simulink model "Model2"  (R2024b)
settings: Solver=ode4  StartTime=0.0  StopTime=100  FixedStep=0.01  RelTol=1e-3
values from neighbouring files (symbols this model uses):
  ARM_P_PID = [10 0 20]*0.1    [Single_ARM_Monte.m]    (also in main_starter.m)
  ARM_T_PID = [100 0 0]    [Single_ARM_Monte.m]    (also in main_starter.m)
  ARM_V_PID = [10 0 5]*0.1    [Single_ARM_Monte.m]    (also in main_starter.m)
  D_Joint0_angle0 = 45    [Single_ARM_Monte.m]    (also in main_starter.m)
  D_Joint0_angle1 = 0    [Single_ARM_Monte.m]    (also in main_starter.m)
  D_Joint0_angle2 = 0    [Single_ARM_Monte.m]    (also in main_starter.m)
  D_Joint0_rate0 = 0    [Single_ARM_Monte.m]    (also in main_starter.m)
  D_Joint0_rate1 = 0    [Single_ARM_Monte.m]    (also in main_starter.m)
  D_Joint0_rate2 = 0    [Single_ARM_Monte.m]    (also in main_starter.m)
  Joint_Motor_Mass = 23    [Single_ARM_Monte.m]    (also in main_starter.m)
  L_Joint0_angle0 = 45    [Single_ARM_Monte.m]    (also in main_starter.m)
  L_Joint0_angle1 = 0    [Single_ARM_Monte.m]    (also in main_starter.m)
  L_Joint0_angle2 = 0    [Single_ARM_Monte.m]    (also in main_starter.m)
  L_Joint0_rate0 = 0    [Single_ARM_Monte.m]    (also in main_starter.m)
  L_Joint0_rate1 = 0    [Single_ARM_Monte.m]    (also in main_starter.m)
  L_Joint0_rate2 = 0    [Single_ARM_Monte.m]    (also in main_starter.m)
  L_Joint_Offset = [ ... (first row only)    [Single_ARM_Monte.m]    (also in main_starter.m)
  Link1_Mass = 11    [Single_ARM_Monte.m]    (also in main_starter.m)
  Link2_Mass = 15.6    [Single_ARM_Monte.m]    (also in main_starter.m)
  Link3_Mass = 11    [Single_ARM_Monte.m]    (also in main_starter.m)
  Motor_transfer_Den = [1 100]    [Single_ARM_Monte.m]    (also in main_starter.m)
  Motor_transfer_Num = [100]    [Single_ARM_Monte.m]    (also in main_starter.m)
  PID_dt = 0.01    [Single_ARM_Monte.m]    (also in main_starter.m)
  R_Joint0_angle0 = 45    [Single_ARM_Monte.m]    (also in main_starter.m)
  R_Joint0_angle1 = 0    [Single_ARM_Monte.m]    (also in main_starter.m)
  R_Joint0_angle2 = 0    [Single_ARM_Monte.m]    (also in main_starter.m)
  R_Joint0_rate0 = 0    [Single_ARM_Monte.m]    (also in main_starter.m)
  R_Joint0_rate1 = 0    [Single_ARM_Monte.m]    (also in main_starter.m)
  R_Joint0_rate2 = 0    [Single_ARM_Monte.m]    (also in main_starter.m)
  RW_Att_D = 0.5    [Single_ARM_Monte.m]    (also in main_starter.m)
  RW_Att_I = 0.2    [Single_ARM_Monte.m]    (also in main_starter.m)
  RW_Att_P = 0.1    [Single_ARM_Monte.m]    (also in main_starter.m)
  RW_Mass = 100    [Single_ARM_Monte.m]    (also in main_starter.m)
  S_Body_Mass = 5    [Single_ARM_Monte.m]    (also in main_starter.m)
  S_init_pos = [0 0 0]'    [Single_ARM_Monte.m]    (also in main_starter.m)
  S_init_vel = [0 0 0]'    [Single_ARM_Monte.m]    (also in main_starter.m)
  T_Body_Mass = 4    [Single_ARM_Monte.m]    (also in main_starter.m)
  T_init_pos = [T_init_pos_list(i,1) T_init_pos_list(i,2) 0]'    [Single_ARM_Monte.m]    (also in main_starter.m = [1 0 0]')
  T_init_vel = [0 0 0]'    [Single_ARM_Monte.m]    (also in main_starter.m)
  Torq_mea_transfer_Den = [1 5]    [Single_ARM_Monte.m]    (also in main_starter.m)
  Torq_mea_transfer_Num = [5]    [Single_ARM_Monte.m]    (also in main_starter.m)
  U_Joint0_angle0 = 45    [Single_ARM_Monte.m]    (also in main_starter.m)
  U_Joint0_angle1 = 0    [Single_ARM_Monte.m]    (also in main_starter.m)
  U_Joint0_angle2 = 0    [Single_ARM_Monte.m]    (also in main_starter.m)
  U_Joint0_rate0 = 0    [Single_ARM_Monte.m]    (also in main_starter.m)
  U_Joint0_rate1 = 0    [Single_ARM_Monte.m]    (also in main_starter.m)
  U_Joint0_rate2 = 0    [Single_ARM_Monte.m]    (also in main_starter.m)
undefined symbols (not defined in the file or in its folder): X, Y, Z
libraries: nesl_utility x315, sm_lib x282, simulink_extras x46, sharedtransform x25, aerolibutil x4, simulink x2, matrix_library x2, dspmtrx3 x1
(part 11 of 12)

== matlab function Model2/Single(Right)_ARM_Simplify/touch ==
  settings: updateMethod=DISCRETE
  data: touch_start input; R_jtc input; R_Jd input; Rv_cmd input; speed_drop_flg output; touch_flg output; q_touch_flg output; speed_drop_vec output
function [speed_drop_flg, touch_flg, q_touch_flg, speed_drop_vec] = detectTouch3(touch_start, R_jtc, R_Jd, Rv_cmd)

    % --- 파라미터 설정 ---

    speed_err_thresh      = 1e-2;
    current_min_thresh    = 0.2e-3;
    current_max_thresh    = 2.5e-1;

    % --- 출력 초기화 ---
    speed_drop_flg  = 0;
    touch_flg       = 0;
    q_touch_flg     = 0;
    speed_drop_vec  = zeros(3,1);  % double 타입 고정

    % --- 전류 추출 ---
    R_qt0 = R_jtc(1);
    R_qt1 = R_jtc(2);
    R_qt2 = R_jtc(3);

    q0_touch_flg = 0;
    q1_touch_flg = 0;
    q2_touch_flg = 0;

    % --- 속도 차이 계산 ---
    raw_vec = abs(Rv_cmd - R_Jd) > speed_err_thresh;
    speed_drop_vec = double(raw_vec);  % 형 변환

    if any(raw_vec)
        speed_drop_flg = 1;
    end

    if touch_start == 1
        if abs(R_qt0) >= current_min_thresh && abs(R_qt0) < current_max_thresh
            q0_touch_flg = 1;
        end
        if abs(R_qt1) >= current_min_thresh && abs(R_qt1) < current_max_thresh
            q1_touch_flg = 1;
        end
        if abs(R_qt2) >= current_min_thresh && abs(R_qt2) < current_max_thresh
            q2_touch_flg = 1;
        end

        if q0_touch_flg || q1_touch_flg || q2_touch_flg
           touch_flg = 1;
        end

        % if  q_touch_flg
        %     touch_flg = 1;
        % end
    end
end

== matlab function Model2/Single(Right)_ARM_Simplify/MATLAB Function16 ==
  settings: updateMethod=DISCRETE
  data: R_J input; R_J_Pos input; R_q input; elapsedTime input; Body_f1 input; Body_f2 input; Body_f3 input; Body_f4 input; Z output; control_mode output; Rv_cmd output; flag_empty_now output; touch_start output; overload_start output; EE_Jaco_start output; system_empty input; system_overload input; system_slip_ing input; system_slip_confirm input; Body_contact output
function [Z,control_mode,Rv_cmd,flag_empty_now,touch_start,overload_start,EE_Jaco_start,Body_contact]  = mlhdlc_fsm_mealy(R_J, R_J_Pos, R_q, elapsedTime, ...
    Body_f1, Body_f2, Body_f3, Body_f4,system_empty,system_overload,system_slip_ing,system_slip_confirm) ...

% system_empty
% define states
S1 = 1; %% pre-grasping
S2 = 2; %% stay
S3 = 3; %% closing (grasping)
S4 = 4; %% regrasping_all
S5 = 5; %% grasp_complete


sub_overload = 11; %% regrasp_empty
sub_empty    = 22; %% regrasp_overload
sub_slip_ing = 33; %% regrasp_slip_ing
sub_slip_conf= 44; %% regrasp_slip_confirm



Rv_cmd = zeros(3,1);
control_mode = zeros(3,1);
flag_empty_now =0;
Z = zeros(1,1);

touch_start=0;
overload_start=0;
empty_start=0;
EE_Jaco_start=0;


% initial_R_condition = [-45 -5 -5];

persistent current_state
if isempty(current_state)
    current_state = 1;
end

persistent slip_latch
if isempty(slip_latch)
    slip_latch = 0;
end

persistent touch_start_flag
if isempty(touch_start_flag)
    touch_start_flag = 0;
end

persistent regrasp_substate
if isempty (regrasp_substate)
    regrasp_substate=0;
end

persistent grip_flg
if isempty(grip_flg)
    grip_flg = 0;
end

Body_contact = (Body_f1 && Body_f2 && Body_f3 && Body_f4) || ...
    (Body_f1 && Body_f3) || (Body_f2 && Body_f4);


%% FSM start

if current_state == S1

    % 
    R_condition_1 = (R_q(1) >= -45-2 && R_q(1) <= -45+2);
    R_condition_2 = (R_q(2) >= -5 && R_q(2) <= 5);
    R_condition_3 = (R_q(3) >= -5 && R_q(3) <= 5);

    R_condition = R_condition_1 && R_condition_2 && R_condition_3;

    condition = R_condition;
    % condition = 1;

    % Rv_cmd = [-45 0 0]'*pi/180;
    Rv_cmd = [-45 0 0]'*pi/180;
    control_mode = [3 3 3]';

    if (condition)
        if trackTime(elapsedTime, condition,1) >= 10
            current_state = 2;

            trackTime(elapsedTime, 0,1);
        end
    else
        current_state = 1;
    end

end

%%%%%%%%%%%%%%%%%%%%%%%%%%%%%%%%%%%%%%%%%%%%%%%%%%%%%%
%%%%%%%%%%%%%%%%%%%%%%%%%%%%%%%%%%%%%%%%%%%%%%%%%%%%%%

if current_state == S2


    if trackTime(elapsedTime, 1, 2) >= 10
        current_state = 3;
        trackTime(elapsedTime, 0, 2);
    else
        current_state = 2;
        Rv_cmd = [0 0 0]'*pi/180;
        control_mode = [2 2 2]';

    end
end

%%%%%%%%%%%%%%%%%%%%%%%%%%%%%%%%%%%%%%%%%%%%%%%%%%%%%%
%%%%%%%%%%%%%%%%%%%%%%%%%%%%%%%%%%%%%%%%%%%%%%%%%%%%%%

if current_state == S3 %% closing

    % Rv_cmd = [0.5 2 1.5]'*1*pi/180;

    Rv_cmd = [1 4 3]'*1*pi/180;
    control_mode = [2 2 2]';
    closing_duration = trackTime(elapsedTime,1,3);


    %%%%%%%%%%%%Predicate 활성화

    overload_start =1;
    empty_start =1;

    if closing_duration >= 5
        touch_start_flag = 1;
    end
    touch_start = touch_start_flag;

    %%%%%%%%%%%%Fail state

    if system_empty ==1 || system_overload==1 || system_slip_ing==1 || system_slip_confirm==1


        if system_empty == 1
            regrasp_substate = sub_empty;

        elseif system_overload == 1
            regrasp_substate = sub_overload;

        elseif system_slip_ing == 1
            regrasp_substate = sub_slip_ing;

        elseif system_slip_confirm == 1
            regrasp_substate = sub_slip_conf;

        end

        current_state = 4;

    end

    %%%%%%%%%%%%%%%%%%%%%%%

    if Body_contact == 1
        grasped_time = trackTime(elapsedTime, 1,4);

        if grasped_time>=1
            current_state = 2;
            trackTime(elapsedTime, 0,4);
        end
    else
        trackTime(elapsedTime, 0,4);
    end

else
    touch_start = 0;

end


%%%%%%%%%%%%%%%%%%%%%%%%%%%%%%%%%%%%%%%%%%%%%%%%%%%%%%
%%%%%%%%%%%%%%%%%%%%%%%%%%%%%%%%%%%%%%%%%%%%%%%%%%%%%%


if current_state == 4

    overload_start =1;
    empty_start =1;
    touch_start =1;
    EE_Jaco_start=1;

    if regrasp_substate == sub_empty

        Rv_cmd = [-1 -2 -1.5]'*pi/180;
        control_mode = [2 2 2]';

        R_condition_1 = (R_q(1) >= -28-2 && R_q(1) <= -28+2);
        R_condition_2 = (R_q(2) >= -2 && R_q(2) <= 2);
        R_condition_3 = (R_q(3) >= -2 && R_q(3) <= 2);

    
        if R_condition_1 && R_condition_2 && R_condition_3
            Rv_cmd = [0 0 0]'*pi/180;
            control_mode = [2 2 2]';
        end

    elseif regrasp_substate == sub_overload

        Rv_cmd = [-0.25 -1 -0.75]'*pi/180;
        control_mode = [2 2 2]';

    elseif regrasp_substate == sub_slip_ing

        Rv_cmd = [0.25 1 0.75]'*pi/180;
        control_mode = [2 2 2]';

        if system_slip_confirm == 1
            slip_latch = 1;  % 한 번이라도 잡히면 latch
        end

        if slip_latch == 1
            Rv_cmd = [-2 -4 -3]'*pi/180;
            control_mode = [2 2 2]';
            % slip_latch = 0;  
        end
        % 
        % elseif system_empty ==1
        %     regrasp_substate =sub_empty;
        % elseif system_overload ==1
        %     regrasp_substate = sub_overload;
        % end


    % elseif regrasp_substate == sub_slip_conf
    % 
    %     Rv_cmd = [-0.25 -1 -0.75]'*pi/180;
    %     control_mode = [2 2 2]';


    else
        Rv_cmd = [-3 -4 -3]';
        control_mode = [2 2 2]';
    end

    if Body_contact == 1
        grasped_time = trackTime(elapsedTime, 1,5);

        if grasped_time>=1
            current_state = 5;
            trackTime(elapsedTime, 0,5);
        end
    else
        trackTime(elapsedTime, 0,5);
    end

    % if some_recovery_condition
    %     current_state = S3;
    %     regrasp_substate = subS_none;
    % end

end


if current_state == 5

    overload_start =1;
  
    %
    % Rv_cmd = [2 4 5]'*pi/180;
    control_mode = [2 2 2]';
    EE = [R_J_Pos(1,4), R_J_Pos(2,4)]';
    EE_ = EE / norm(EE);

    Rv_cmd = [0 0 0]';
    

    if Body_contact == 1


        if grip_flg == 0
            grip_flg = 1;
            v_cmd = [-0.01; 0.0] .* EE_;
            R_Jacob = jacobian_3link(R_J);
            Rv_cmd = pinv(R_Jacob) * v_cmd;
        else
            Rv_cmd = [-2; -4; -3] * pi/180;
        end

        if (grip_flg == 1)
            v_cmd = [-0.01, 0.0]'.*EE_;
            R_Jacob = jacobian_3link(R_J);
            Rv_cmd = pinv(R_Jacob)*v_cmd;
        end

        % if system_overload == 1
        %     Rv_cmd = [-1; -2; -1];
        %     control_mode = [2 2 2]';
        %     return;
        % end

    end

   
end

  Z = current_state;

end


function J = jacobian_3link(theta)
% 링크 길이
L1 = 0.2;
L2 = 0.15;
L3 = 0.1;

t1 = theta(1);
t2 = theta(2);
t3 = theta(3);

t12 = t1 + t2;
t123 = t12 + t3;

% 자코비안 계산
J = zeros(2, 3);

J(1,1) = -L1*sin(t1) - L2*sin(t12) - L3*sin(t123);
J(1,2) =           - L2*sin(t12) - L3*sin(t123);
J(1,3) =                         - L3*sin(t123);

J(2,1) =  L1*cos(t1) + L2*cos(t12) + L3*cos(t123);
J(2,2) =             L2*cos(t12) + L3*cos(t123);
J(2,3) =                         L3*cos(t123);
end



function [temp] = trackTime(elapsedTime, timer_flg, id)
persistent isTiming startTime totalDuration
temp = 0;

if isempty(isTiming)
    isTiming = false(10,1);  % 최대 10개의 타이머 ID 지원
    startTime = zeros(10,1);
    totalDuration = zeros(10,1);
end


if timer_flg == 1 && ~isTiming(id)
    startTime(id) = elapsedTime;
    isTiming(id) = true;


elseif timer_flg == 1 && isTiming(id)
    currentDuration = elapsedTime - startTime(id);
    temp = currentDuration;


elseif timer_flg == 0 && isTiming(id)
    totalDuration(id) = elapsedTime - startTime(id);

    isTiming(id) = false;
    startTime(id) = 0;
    totalDuration(id) = 0;
end
end


%%%%%%%%%%%%%%

== matlab function Model2/Single_ARM/MATLAB Function5 ==
  data: v_sig input; v_out output; vd_out output; vd_sig input; t_mea input
function [v_out, vd_out] = limit_checker(v_sig,vd_sig,  t_mea)


if(abs(t_mea)>=0.5)
    vd_out = 0;
    v_out = 0;
else
    vd_out = vd_sig;
    v_out = v_sig;
end




end

== matlab function Model2/Single_ARM/MATLAB Function6 ==
  settings: updateMethod=DISCRETE
  data: cmd input; t_cmd output; cmd_d input; t_mea input; vd_mea input; v_mea input; p_mea input; mode input; tc_gain input; vc_gain input; pc_gain input; dt input
function t_cmd = motor_control(cmd,cmd_d, t_mea, vd_mea, v_mea, p_mea, mode, tc_gain, vc_gain, pc_gain, dt)

persistent I_save
persistent first_flg

if isempty(first_flg)
    I_save = 0;
    first_flg = 1;
end

if(mode == 1)%torque control
    % cmd : torque command [Nm]
    kp = tc_gain(1);
    ki = tc_gain(2);
    err = cmd - t_mea;
    t_cmd = kp*(cmd - t_mea) + ki*I_save;
    I_save = I_save + err*dt;

elseif(mode == 2) %velocity control
    % cmd : velocity command [rad/s]
    kp = vc_gain(1);
    % ki = vc_gain(2);
    kd = vc_gain(3);

    err = cmd - v_mea;
    errd = cmd_d - vd_mea;
    % t_cmd = (kp*err) + (kd*errd);
    t_cmd = (kp*err) + (kd*errd);
elseif(mode == 3) %position control : position command [rad]
    kp = pc_gain(1);
    % ki = pc_gain(2);
    kd = pc_gain(3);

    err = cmd - p_mea;
    errd = cmd_d - v_mea;
    t_cmd = (kp*err) + (kd*errd);
else%torque control
    t_cmd = 0;
end



end

== matlab function Model2/Single_ARM/MATLAB Function7 ==
  data: v_sig input; v_out output; vd_out output; vd_sig input; t_mea input
function [v_out, vd_out] = limit_checker(v_sig,vd_sig,  t_mea)


if(abs(t_mea)>=0.5)
    vd_out = 0;
    v_out = 0;
else
    vd_out = vd_sig;
    v_out = v_sig;
end




end

== matlab function Model2/Single(Right)_ARM_Simplify/slip_kinematics ==
  data: EE_vel_t output; EE_vel_J input; slip_kinematics output; EE_vel_J_pre input; EE_Jaco_start input
function [EE_vel_t,slip_kinematics]  = kinema_slip(EE_vel_J,EE_vel_J_pre,EE_Jaco_start)

    vel_min = -0.005;
    vel_max = 0.005;
    
    dvel_min = -0.005;
    dvel_max = 5e-03;
    
    dt= 3;
    
    dEE_vel = EE_vel_J_pre-EE_vel_J;
    EE_vel_t = dEE_vel/dt;
    
    if EE_Jaco_start==1 && all(EE_vel_J >= vel_min & EE_vel_J <= vel_max) && all(EE_vel_t<=dvel_max)
        slip_kinematics =1;
    else
        slip_kinematics=0;
    
    end

end

%%

== matlab function Model2/Single(Right)_ARM_Simplify/MATLAB Function1 ==
  data: u input; y output
function y = fcn(u)

y = u(:,3);

end

== matlab function Model2/Quad_ARM_Simplify/Mount_Frame_Based_Jacobian_Test/MATLAB Function4 ==
  data: u input; y output
function y = fcn(u)

y = u(:,4);

end

== matlab function Model2/Quad_ARM_Simplify/Mount_Frame_Based_Jacobian_Test/Right_ARM_Real_Simple_FK ==
  data: theta input; positions output; ee_pose output
function [positions, ee_pose] = fk_R_3link_simplify(theta)
    % theta: [theta1, theta2, theta3] (rad)
    % a1, a2, a3: 링크 길이
    % positions: [P0; P1; P2; P3] (각 조인트 위치)
    % ee_pose: [x, y, phi] (EE 위치 + 자세)
    % L0 = 0.04494;
    % L1 = 0.08979;
    % L2 = 0.1665;
    % L3a = 0.02945;
    % L3b = 0.1232;


    offset0 = -atan2(0.04494, 0.08979);
    offset1 = +atan2(0.04494, 0.08979);
    offset2 = -atan2(0.02945, 0.1232);
    offset = 1*[offset0,offset1,offset2]';

    theta = theta + offset;

    L = [sqrt(0.04494^2 + 0.08979^2);
           0.1665;
           sqrt(0.02945^2 + 0.1232^2)];

    theta1 = theta(1);
    theta2 = theta(2);
    theta3 = theta(3);

    % 누적 각도
    t1 = theta1;
    t2 = theta1 + theta2;
    t3 = t2 + theta3;

    % 각 조인트 위치 계산
    P0 = [0; 0];
    P1 = P0 + L(1) * [cos(t1); sin(t1)];
    P2 = P1 + L(2) * [cos(t2); sin(t2)];
    P3 = P2 + L(3) * [cos(t3); sin(t3)];

    % 자세
    phi = t3;

    % 출력
    positions = [P0, P1, P2, P3];  % 각 열이 각 위치
    ee_pose = [P3(1), P3(2)]'; % EE 위치 및 방향
end

== matlab function Model2/Quad_ARM_Simplify/Right_ARM_Real_FK ==
  data: theta input; positions output; ee_pose output
function [positions, ee_pose] = fk_R_3link_explicit(theta)
    L0 = 0.04494;
    L1 = 0.08979;
    L2 = 0.1665;
    L3a = 0.02945;
    L3b = 0.1232;

    t0 = theta(1);
    t1 = theta(2);
    t2 = theta(3);
    t01 = t0 + t1;
    t012 = t01 + t2;

    R = @(theta) [-cos(theta); -sin(theta)];

    P0 = [0; 0];
    P1 = P0 - L0 * R(t0 - pi/2);
    P2 = P1 - L1 * R(t0);
    P3 = P2 - L2 * R(t01);
    P4 = P3 - L3a * R(t012 - pi/2);
    ee_pose = P4 - L3b * R(t012);  % EE 위치
    positions = [P1,P2,P3,P4,ee_pose];
end

== matlab function Model2/Quad_ARM_Simplify/Right_ARM_Real_Simple_FK ==
  data: theta input; positions output; ee_pose output
function [positions, ee_pose] = fk_R_3link_simplify(theta)
    % theta: [theta1, theta2, theta3] (rad)
    % a1, a2, a3: 링크 길이
    % positions: [P0; P1; P2; P3] (각 조인트 위치)
    % ee_pose: [x, y, phi] (EE 위치 + 자세)
    % L0 = 0.04494;
    % L1 = 0.08979;
    % L2 = 0.1665;
    % L3a = 0.02945;
    % L3b = 0.1232;


    offset0 = -atan2(0.04494, 0.08979);
    offset1 = +atan2(0.04494, 0.08979);
    offset2 = -atan2(0.02945, 0.1232);
    offset = 1*[offset0,offset1,offset2]';

    theta = theta + offset;

    L = [sqrt(0.04494^2 + 0.08979^2);
           0.1665;
           sqrt(0.02945^2 + 0.1232^2)];

    theta1 = theta(1);
    theta2 = theta(2);
    theta3 = theta(3);

    % 누적 각도
    t1 = theta1;
    t2 = theta1 + theta2;
    t3 = t2 + theta3;

    % 각 조인트 위치 계산
    P0 = [0; 0];
    P1 = P0 + L(1) * [cos(t1); sin(t1)];
    P2 = P1 + L(2) * [cos(t2); sin(t2)];
    P3 = P2 + L(3) * [cos(t3); sin(t3)];

    % 자세
    phi = t3;

    % 출력
    positions = [P0, P1, P2, P3];  % 각 열이 각 위치
    ee_pose = [P3(1), P3(2)]'; % EE 위치 및 방향
end

== matlab function Model2/Quad_ARM_Simplify/MATLAB Function4 ==
  data: u input; y output
function y = fcn(u)

y = u(:,4);

end

== matlab function Model2/Quad_ARM_Simplify/Mount_Frame_Based_Jacobian_Test/Right_ARM_Jacobian ==
  data: theta input; J output
function J = jacobian_fk_R_3link_explicit(theta)
    % 링크 길이
    L0 = 0.04494;
    L1 = 0.08979;
    L2 = 0.1665;
    L3a = 0.02945;
    L3b = 0.1232;

    % 조인트 각도
    t0 = theta(1);
    t1 = theta(2);
    t2 = theta(3);

    t01 = t0 + t1;
    t012 = t01 + t2;

    % 편미분 벡터 함수 dR = d/dθ of R(θ)
    dR = @(theta) [sin(theta); -cos(theta)];

    % ∂x/∂theta1
    J1 = ...
        L0 * dR(t0 - pi/2) + ...
        L1 * dR(t0) + ...
        L2 * dR(t01) + ...
        L3a * dR(t012 - pi/2) + ...
        L3b * dR(t012);

    % ∂x/∂theta2
    J2 = ...
        L2 * dR(t01) + ...
        L3a * dR(t012 - pi/2) + ...
        L3b * dR(t012);

    % ∂x/∂theta3
    J3 = ...
        L3a * dR(t012 - pi/2) + ...
        L3b * dR(t012);

    % 최종 자코비안
    J = [J1, J2, J3];
end

== matlab function Model2/Single(Right)_ARM_Simplify/Jacobian_based_EE_Control(Rate) ==
  data: q input; qd_cmd output; target_pos input
function qd_cmd = Jacobian_based_EE_Control(q, target_pos)
% target_pos = [0.3 0 0]';
pos = fk_3link_explicit(q);
J = jacobian_3link(q);

L = ...
[sqrt(0.04494^2 + 0.08979^2);
 0.1665;
 sqrt(0.02945^2 + 0.1232^2)];

% 목표 거리
total_length = sum(L);
if norm(target_pos) > total_length
    % error("목표가 작업공간을 벗어났습니다.");
    target_pos = total_length*(target_pos/norm(target_pos));
end

err = 2*(target_pos - pos);
Z = 0*[1 1 1]';
qd_cmd = pinv(J)*err + (eye(3,3) - pinv(J)*J)*Z;

end

function pos = fk_3link_explicit(theta)
    L0 = 0.04494;
    L1 = 0.08979;
    L2 = 0.1665;
    L3a = 0.02945;
    L3b = 0.1232;

    t0 = theta(1);
    t1 = theta(2);
    t2 = theta(3);
    t01 = t0 + t1;
    t012 = t01 + t2;

    R = @(theta) [cos(theta); sin(theta)];

    P0 = [0; 0];
    P1 = P0 + L0 * R(t0 + pi/2);
    P2 = P1 + L1 * R(t0);
    P3 = P2 + L2 * R(t01);
    P4 = P3 + L3a * R(t012 + pi/2);
    pos = P4 + L3b * R(t012);  % EE 위치
end

function J = jacobian_3link(theta)
    L0 = 0.04494;
    L1 = 0.08979;
    L2 = 0.1665;
    L3a = 0.02945;
    L3b = 0.1232;

    t0 = theta(1);
    t1 = theta(2);
    t2 = theta(3);
    t01 = t0 + t1;
    t012 = t01 + t2;

    Rp = @(theta) [-sin(theta); cos(theta)]; 

    J1 =  L0 * Rp(t0 + pi/2) ...
         +L1 * Rp(t0) ...
         +L2 * Rp(t01) ...
         +L3a * Rp(t012 + pi/2) ...
         +L3b * Rp(t012);

    J2 =  L2 * Rp(t01) ...
         +L3a * Rp(t012 + pi/2) ...
         +L3b * Rp(t012);

    J3 =  L3a * Rp(t012 + pi/2) ...
         +L3b * Rp(t012);

    J = [J1, J2, J3];
end

== matlab function Model2/Single(Right)_ARM_Simplify/Fabrik_based_EE_Control(Angle) ==
  data: target input; q_list output; tol input; pos_list output; max_iter input; iter_fin output
function [q_list, pos_list, iter_fin] = fabrik_3link(target, tol, max_iter)
% target: [x; y] 목표 위치
% L: [L1, L2, L3] 링크 길이
% tol: 허용 오차 (예: 1e-4)
% max_iter: 반복 한계 (예: 100)

L = ...
[sqrt(0.04494^2 + 0.08979^2);
 0.1665;
 sqrt(0.02945^2 + 0.1232^2)];


[positions, ee_pose] = fk_3link([50,0,0]'*pi/180, L(1), L(2), L(3));

% 초기 관절 위치 (x, y) 초기화
pos_list = zeros(2, 4); % P0, P1, P2, P3
pos_list(:,1) = [0; 0];                    % Base
pos_list(:,2) = positions(:,1) + [L(1); 0]; % P1
pos_list(:,3) = positions(:,2) + [L(2); 0]; % P2
pos_list(:,4) = positions(:,3) + [L(3); 0]; % EE (초기화)

% Base 저장
base = pos_list(:,1);

% 목표 거리
total_length = sum(L);
if norm(target - base) > total_length
    % error("목표가 작업공간을 벗어났습니다.");
    target = total_length*(target/norm(target));
end

iter_fin = 0;

for iter = 1:max_iter
    % 1. FORWARD REACHING
    pos_list(:,4) = target; % 끝단 고정
    for i = 3:-1:1
        r = norm(pos_list(:,i+1) - pos_list(:,i));
        lambda = L(i) / r;
        pos_list(:,i) = (1 - lambda) * pos_list(:,i+1) + lambda * pos_list(:,i);
    end

    % 2. BACKWARD REACHING
    pos_list(:,1) = base; % base 고정
    for i = 1:3
        r = norm(pos_list(:,i+1) - pos_list(:,i));
        lambda = L(i) / r;
        pos_list(:,i+1) = (1 - lambda) * pos_list(:,i) + lambda * pos_list(:,i+1);
    end

    % 3. 수렴 확인
    err = norm(pos_list(:,end) - target);
    if err < tol
        break;
    end
    iter_fin = iter;
end

% P0 = joint_pos(:,1); P1 = joint_pos(:,2);
P2 = pos_list(:,2); P3 = pos_list(:,3);
% P4 = joint_pos(:,5); 
P5 = pos_list(:,4);

t0 = atan2(P2(2), P2(1));
temp = P3 - P2;
t1 = atan2(temp(2), temp(1)) - t0;
temp = P5 - P3;
t2 = atan2(temp(2), temp(1)) - t0 - t1;



q_list = [t0,t1,t2]';

end

function [positions, ee_pose] = fk_3link(theta, a1, a2, a3)
    % theta: [theta1, theta2, theta3] (rad)
    % a1, a2, a3: 링크 길이
    % positions: [P0; P1; P2; P3] (각 조인트 위치)
    % ee_pose: [x, y, phi] (EE 위치 + 자세)

    theta1 = theta(1);
    theta2 = theta(2);
    theta3 = theta(3);

    % 누적 각도
    t1 = theta1;
    t2 = theta1 + theta2;
    t3 = t2 + theta3;

    % 각 조인트 위치 계산
    P0 = [0; 0];
    P1 = P0 + a1 * [cos(t1); sin(t1)];
    P2 = P1 + a2 * [cos(t2); sin(t2)];
    P3 = P2 + a3 * [cos(t3); sin(t3)];

    % 자세
    phi = t3;

    % 출력
    positions = [P0, P1, P2, P3];  % 각 열이 각 위치
    ee_pose = [P3(1), P3(2)]'; % EE 위치 및 방향
end

== matlab function Model2/Single(Right)_ARM_Simplify/slip_kinematics_current ==
  data: slip_kine_flg input; slip_dual_flg output; slip_warning_flg input; slip_dual_flg_pre input
function slip_dual_flg = dual_slip(slip_kine_flg,slip_warning_flg,slip_dual_flg_pre)

    
    if slip_kine_flg==1 && slip_warning_flg==1
    
        slip_dual_flg=1;
    else
        slip_dual_flg=0;
    
    end

    dslip_flg = slip_dual_flg_pre-slip_dual_flg;

    if dslip_flg 





end

== matlab function Model2/Single(Right)_ARM_Simplify/MATLAB Function5 ==
  data: theta input; pos output
function pos = fk_3link_explicit(theta)
    L0 = 0.04494;
    L1 = 0.08979;
    L2 = 0.1665;
    L3a = 0.02945;
    L3b = 0.1232;

    t0 = theta(1);
    t1 = theta(2);
    t2 = theta(3);
    t01 = t0 + t1;
    t012 = t01 + t2;

    R = @(theta) [cos(theta); sin(theta)];

    P0 = [0; 0];
    P1 = P0 + L0 * R(t0 + pi/2);
    P2 = P1 + L1 * R(t0);
    P3 = P2 + L2 * R(t01);
    P4 = P3 + L3a * R(t012 + pi/2);
    pos = P4 + L3b * R(t012);  % EE 위치
end

== matlab function Model2/Single(Right)_ARM_Simplify/MATLAB Function6 ==
  data: theta input; positions output; ee_pose output
function [positions, ee_pose] = fk_3link_simplify(theta)
    % theta: [theta1, theta2, theta3] (rad)
    % a1, a2, a3: 링크 길이
    % positions: [P0; P1; P2; P3] (각 조인트 위치)
    % ee_pose: [x, y, phi] (EE 위치 + 자세)

    L = [sqrt(0.04494^2 + 0.08979^2);
           0.1665;
           sqrt(0.02945^2 + 0.1232^2)];

    theta1 = theta(1);
    theta2 = theta(2);
    theta3 = theta(3);

    % 누적 각도
    t1 = theta1;
    t2 = theta1 + theta2;
    t3 = t2 + theta3;

    % 각 조인트 위치 계산
    P0 = [0; 0];
    P1 = P0 + L(1) * [cos(t1); sin(t1)];
    P2 = P1 + L(2) * [cos(t2); sin(t2)];
    P3 = P2 + L(3) * [cos(t3); sin(t3)];

    % 자세
    phi = t3;

    % 출력
    positions = [P0, P1, P2, P3];  % 각 열이 각 위치
    ee_pose = [P3(1), P3(2)]'; % EE 위치 및 방향
end

== matlab function Model2/Single(Right)_ARM_Simplify/MATLAB Function2 ==
  data: u input; y output
function y = fcn(u)

y = u(:,4);

end

== matlab function Model2/Quad_ARM_Simplify/Mount_Frame_Based_Jacobian_Test/Right_ARM_Real_FK ==
  data: theta input; positions output; ee_pose output
function [positions, ee_pose] = fk_R_3link_explicit(theta)
    L0 = 0.04494;
    L1 = 0.08979;
    L2 = 0.1665;
    L3a = 0.02945;
    L3b = 0.1232;

    t0 = theta(1);
    t1 = theta(2);
    t2 = theta(3);
    t01 = t0 + t1;
    t012 = t01 + t2;

    R = @(theta) [-cos(theta); -sin(theta)];

    P0 = [0; 0];
    P1 = P0 - L0 * R(t0 - pi/2);
    P2 = P1 - L1 * R(t0);
    P3 = P2 - L2 * R(t01);
    P4 = P3 - L3a * R(t012 - pi/2);
    ee_pose = P4 - L3b * R(t012);  % EE 위치
    positions = [P1,P2,P3,P4,ee_pose];
end

== matlab function Model2/Single(Right)_ARM_Simplify/Openning_Motion_Sequence1 ==
  data: t input; res output; mode output
function [res, mode] = Motion_CMD(t)

deg2rad = pi/180;

if (t <= 10)
    res = [45 -90 -180]'*deg2rad;

elseif ((t>=10) && (t<=20))
    res = [45 0 -180]'*deg2rad;
else
    res = [45 0 0]'*deg2rad;
end

mode = [3 3 3]';

end

== matlab function Model2/Single(Right)_ARM_Simplify/Right_ARM/MATLAB Function2 ==
  settings: updateMethod=DISCRETE
  data: cmd input; t_cmd output; cmd_d input; t_mea input; vd_mea input; v_mea input; p_mea input; mode input; tc_gain input; vc_gain input; pc_gain input; dt input
function t_cmd = motor_control(cmd, cmd_d, t_mea, vd_mea, v_mea, p_mea, mode, tc_gain, vc_gain, pc_gain, dt)

persistent I_save
persistent first_flg

if isempty(first_flg)
    I_save = 0;
    first_flg = 1;
end

if(mode == 1)%torque control
    % cmd : torque command [Nm]
    kp = tc_gain(1);
    ki = tc_gain(2);
    err = cmd - t_mea;
    t_cmd = kp*(cmd - t_mea) + ki*I_save;
    I_save = I_save + err*dt;

elseif(mode == 2) %velocity control
    % cmd : velocity command [rad/s]
    kp = vc_gain(1);
    % ki = vc_gain(2);
    kd = vc_gain(3);

    err = cmd - v_mea;
    errd = cmd_d - vd_mea;
    % t_cmd = (kp*err) + (kd*errd);
    t_cmd = (kp*err) + (kd*errd);
elseif(mode == 3) %position control : position command [rad]
    kp = pc_gain(1);
    % ki = pc_gain(2);
    kd = pc_gain(3);

    err = cmd - p_mea;
    errd = cmd_d - v_mea;
    t_cmd = (kp*err) + (kd*errd);
else%torque control
    t_cmd = 0;
end



end

== matlab function Model2/Single(Right)_ARM_Simplify/Right_ARM/MATLAB Function3 ==
  data: v_sig input; v_out output; vd_out output; vd_sig input; t_mea input
function [v_out, vd_out] = limit_checker(v_sig,vd_sig,  t_mea)


if(abs(t_mea)>=0.001)
    vd_out = 0;
    v_out = 0;
else
    vd_out = vd_sig;
    v_out = v_sig;
end




end

== matlab function Model2/Single(Right)_ARM_Simplify/Right_ARM/MATLAB Function4 ==
  settings: updateMethod=DISCRETE
  data: cmd input; t_cmd output; cmd_d input; t_mea input; vd_mea input; v_mea input; p_mea input; mode input; tc_gain input; vc_gain input; pc_gain input; dt input
function t_cmd = motor_control(cmd,cmd_d, t_mea, vd_mea, v_mea, p_mea, mode, tc_gain, vc_gain, pc_gain, dt)

persistent I_save
persistent first_flg

if isempty(first_flg)
    I_save = 0;
    first_flg = 1;
end

if(mode == 1)%torque control
    % cmd : torque command [Nm]
    kp = tc_gain(1);
    ki = tc_gain(2);
    err = cmd - t_mea;
    t_cmd = kp*(cmd - t_mea) + ki*I_save;
    I_save = I_save + err*dt;

elseif(mode == 2) %velocity control
    % cmd : velocity command [rad/s]
    kp = vc_gain(1);
    % ki = vc_gain(2);
    kd = vc_gain(3);

    err = cmd - v_mea;
    errd = cmd_d - vd_mea;
    % t_cmd = (kp*err) + (kd*errd);
    t_cmd = (kp*err) + (kd*errd);
elseif(mode == 3) %position control : position command [rad]
    kp = pc_gain(1);
    ki = pc_gain(2);
    kd = pc_gain(3);

    err = cmd - p_mea;
    errd = cmd_d - v_mea;
    t_cmd = (kp*err) + (kd*errd);
else%torque control
    t_cmd = 0;
end



end

== matlab function Model2/Single(Right)_ARM_Simplify/Right_ARM/MATLAB Function5 ==
  data: v_sig input; v_out output; vd_out output; vd_sig input; t_mea input
function [v_out, vd_out] = limit_checker(v_sig,vd_sig,  t_mea)


if(abs(t_mea)>=0.001)
    vd_out = 0;
    v_out = 0;
else
    vd_out = vd_sig;
    v_out = v_sig;
end




end

== matlab function Model2/Single(Right)_ARM_Simplify/Right_ARM/MATLAB Function6 ==
  settings: updateMethod=DISCRETE
  data: cmd input; t_cmd output; cmd_d input; t_mea input; vd_mea input; v_mea input; p_mea input; mode input; tc_gain input; vc_gain input; pc_gain input; dt input
function t_cmd = motor_control(cmd,cmd_d, t_mea, vd_mea, v_mea, p_mea, mode, tc_gain, vc_gain, pc_gain, dt)

persistent I_save
persistent first_flg

if isempty(first_flg)
    I_save = 0;
    first_flg = 1;
end

if(mode == 1)%torque control
    % cmd : torque command [Nm]
    kp = tc_gain(1);
    ki = tc_gain(2);
    err = cmd - t_mea;
    t_cmd = kp*(cmd - t_mea) + ki*I_save;
    I_save = I_save + err*dt;

elseif(mode == 2) %velocity control
    % cmd : velocity command [rad/s]
    kp = vc_gain(1);
    % ki = vc_gain(2);
    kd = vc_gain(3);

    err = cmd - v_mea;
    errd = cmd_d - vd_mea;
    % t_cmd = (kp*err) + (kd*errd);
    t_cmd = (kp*err) + (kd*errd);
elseif(mode == 3) %position control : position command [rad]
    kp = pc_gain(1);
    % ki = pc_gain(2);
    kd = pc_gain(3);

    err = cmd - p_mea;
    errd = cmd_d - v_mea;
    t_cmd = (kp*err) + (kd*errd);
else%torque control
    t_cmd = 0;
end



end

== matlab function Model2/Single(Right)_ARM_Simplify/Right_ARM/MATLAB Function7 ==
  data: v_sig input; v_out output; vd_out output; vd_sig input; t_mea input
function [v_out, vd_out] = limit_checker(v_sig,vd_sig,  t_mea)


if(abs(t_mea)>=0.001)
    vd_out = 0;
    v_out = 0;
else
    vd_out = vd_sig;
    v_out = v_sig;
end




end

== matlab function Model2/Single(Right)_ARM_Simplify/slip_kinematics+Timer ==
  settings: updateMethod=DISCRETE
  data: EE_vel_t output; EE_vel_J input; slip_kinematics output; EE_Jaco_start input; elapsedTime input
function [EE_vel_t,slip_kinematics]  = kinema_slip(EE_vel_J,EE_Jaco_start,elapsedTime)


    persistent EE_vel_J_pre lastTime
    if isempty(EE_vel_J_pre)
        EE_vel_J_pre=[0 0]';
        lastTime = elapsedTime;
    end
    
    dt = elapsedTime - lastTime;
 
    vel_min = -0.005;
    vel_max = 0.005;
    
    dvel_min = -0.005;
    dvel_max = 5e-03;
   

    dEE_vel = EE_vel_J_pre-EE_vel_J;

    EE_vel_t = dEE_vel/dt;
    
    if EE_Jaco_start==1 && all(EE_vel_J >= vel_min & EE_vel_J <= vel_max) && all(EE_vel_t<=dvel_max)
        slip_kinematics =1;
    else
        slip_kinematics=0;
    
    end

    if trackTime(elapsedTime, 1) == 1
        EE_vel_J_pre = EE_vel_J;
        lastTime = elapsedTime;
    end

end

%%
function temp = trackTime(elapsedTime, timer_flg)
    persistent isTiming startTime

    temp = 0;
    duration_time= 3; %[sec]
    
    if isempty(isTiming)
        isTiming = 0;
        startTime = 0;
    end

    if timer_flg == 1
        if isTiming == 0
            startTime = elapsedTime;
            isTiming = 1;
        else
            if elapsedTime - startTime >= duration_time
                temp = duration_time;
                startTime = elapsedTime;  % 타이머 리셋해서 다음 1초 기다림
            end
        end
    else
        isTiming = 0;
        startTime = 0;
    end
end

== matlab function Model2/Quad_ARM_Simplify/Mount_Frame_Based_Jacobian_Test/MATLAB Function3 ==
  data: u input; y output
function y = fcn(u)

y = u(:,4);

end

== matlab function Model2/Quad_ARM_Simplify/Mount_Frame_Based_Jacobian_Test/MATLAB Function7 ==
  data: u input; y output
function y = fcn(u)

y = u(:,4);

end

== matlab function Model2/Quad_ARM_Simplify/Mount_Frame_Based_Jacobian_Test/MATLAB Function8 ==
  data: u input; y output
function y = fcn(u)

y = u(:,4);

end

== matlab function Model2/Quad_ARM_Simplify/Mount_Frame_Based_Jacobian_Test/Right_ARM_Jacobian1 ==
  data: theta input; J output
function J = jacobian_fk_R_3link_explicit(theta)
    % 링크 길이
    L0 = 0.04494;
    L1 = 0.08979;
    L2 = 0.1665;
    L3a = 0.02945;
    L3b = 0.1232;

    % 조인트 각도
    t0 = theta(1);
    t1 = theta(2);
    t2 = theta(3);

    t01 = t0 + t1;
    t012 = t01 + t2;

    % 편미분 벡터 함수 dR = d/dθ of R(θ)
    dR = @(theta) [sin(theta); -cos(theta)];

    % ∂x/∂theta1
    J1 = ...
        L0 * dR(t0 - pi/2) + ...
        L1 * dR(t0) + ...
        L2 * dR(t01) + ...
        L3a * dR(t012 - pi/2) + ...
        L3b * dR(t012);

    % ∂x/∂theta2
    J2 = ...
        L2 * dR(t01) + ...
        L3a * dR(t012 - pi/2) + ...
        L3b * dR(t012);

    % ∂x/∂theta3
    J3 = ...
        L3a * dR(t012 - pi/2) + ...
        L3b * dR(t012);

    % 최종 자코비안
    J = [J1, J2, J3];
end

== matlab function Model2/Quad_ARM_Simplify/Mount_Frame_Based_Jacobian_Test/Right_ARM_Real_FK1 ==
  data: theta input; positions output; ee_pose output
function [positions, ee_pose] = fk_R_3link_explicit(theta)
    L0 = 0.04494;
    L1 = 0.08979;
    L2 = 0.1665;
    L3a = 0.02945;
    L3b = 0.1232;

    t0 = theta(1);
    t1 = theta(2);
    t2 = theta(3);
    t01 = t0 + t1;
    t012 = t01 + t2;

    R = @(theta) [-cos(theta); -sin(theta)];

    P0 = [0; 0];
    P1 = P0 - L0 * R(t0 - pi/2);
    P2 = P1 - L1 * R(t0);
    P3 = P2 - L2 * R(t01);
    P4 = P3 - L3a * R(t012 - pi/2);
    ee_pose = P4 - L3b * R(t012);  % EE 위치
    positions = [P1,P2,P3,P4,ee_pose];
end

== matlab function Model2/Quad_ARM_Simplify/Mount_Frame_Based_Jacobian_Test/Right_ARM_Real_Simple_FK1 ==
  data: theta input; positions output; ee_pose output
function [positions, ee_pose] = fk_R_3link_simplify(theta)
    % theta: [theta1, theta2, theta3] (rad)
    % a1, a2, a3: 링크 길이
    % positions: [P0; P1; P2; P3] (각 조인트 위치)
    % ee_pose: [x, y, phi] (EE 위치 + 자세)
    % L0 = 0.04494;
    % L1 = 0.08979;
    % L2 = 0.1665;
    % L3a = 0.02945;
    % L3b = 0.1232;


    offset0 = -atan2(0.04494, 0.08979);
    offset1 = +atan2(0.04494, 0.08979);
    offset2 = -atan2(0.02945, 0.1232);
    offset = 1*[offset0,offset1,offset2]';

    theta = theta + offset;

    L = [sqrt(0.04494^2 + 0.08979^2);
           0.1665;
           sqrt(0.02945^2 + 0.1232^2)];

    theta1 = theta(1);
    theta2 = theta(2);
    theta3 = theta(3);

    % 누적 각도
    t1 = theta1;
    t2 = theta1 + theta2;
    t3 = t2 + theta3;

    % 각 조인트 위치 계산
    P0 = [0; 0];
    P1 = P0 + L(1) * [cos(t1); sin(t1)];
    P2 = P1 + L(2) * [cos(t2); sin(t2)];
    P3 = P2 + L(3) * [cos(t3); sin(t3)];

    % 자세
    phi = t3;

    % 출력
    positions = [P0, P1, P2, P3];  % 각 열이 각 위치
    ee_pose = [P3(1), P3(2)]'; % EE 위치 및 방향
end

== matlab function Model2/Single(Right)_ARM_Simplify/MATLAB Function ==
  settings: updateMethod=DISCRETE
  data: dTime output; elapsedTime input; differ_input output; input input
function [dTime, differ_input] = ex(elapsedTime, input)
    
    persistent pre_input 
    if isempty(pre_input)
        pre_input=0;
    end

    persistent pre_time 
    if isempty(pre_time)
        pre_time=0;
    end

    dTime=0;


    if trackTime(elapsedTime,1) ==3
        pre_input = input;
        pre_time=elapsedTime;
        % dTime = elapsedTime - pre_time;
        % dTime = 3;
    end

    dTime = elapsedTime - pre_time;

    differ_input = (input - pre_input)/dTime;
end





function temp = trackTime(elapsedTime, timer_flg)
    persistent isTiming startTime

    temp = 0;
    duration_time= 3; %[sec]
    
    if isempty(isTiming)
        isTiming = 0;
        startTime = 0;
    end

    if timer_flg == 1
        if isTiming == 0
            startTime = elapsedTime;
            isTiming = 1;
        else
            if elapsedTime - startTime >= duration_time
                temp = duration_time;
                startTime = elapsedTime; 
            end
        end
    else
        isTiming = 0;
        startTime = 0;
    end
end

== matlab function Model2/Single(Right)_ARM_Simplify/MATLAB Function3 ==
  data: u input; y output
function y = fcn(u)

y = u(:,4);

end

== matlab function Model2/Single(Right)_ARM_Simplify/MATLAB Function4 ==
  data: u input; y output
function y = fcn(u)

y = u(:,4);

end

== matlab function Model2/Single(Right)_ARM_Simplify/Right_ARM_Jacobian ==
  data: theta input; J output
function J = jacobian_fk_R_3link_explicit(theta)
    % 링크 길이
    L0 = 0.04494;
    L1 = 0.08979;
    L2 = 0.1665;
    L3a = 0.02945;
    L3b = 0.1232;

    % 조인트 각도
    t0 = theta(1);
    t1 = theta(2);
    t2 = theta(3);

    t01 = t0 + t1;
    t012 = t01 + t2;

    % 편미분 벡터 함수 dR = d/dθ of R(θ)
    dR = @(theta) [sin(theta); -cos(theta)];

    % ∂x/∂theta1
    J1 = ...
        L0 * dR(t0 - pi/2) + ...
        L1 * dR(t0) + ...
        L2 * dR(t01) + ...
        L3a * dR(t012 - pi/2) + ...
        L3b * dR(t012);

    % ∂x/∂theta2
    J2 = ...
        L2 * dR(t01) + ...
        L3a * dR(t012 - pi/2) + ...
        L3b * dR(t012);

    % ∂x/∂theta3
    J3 = ...
        L3a * dR(t012 - pi/2) + ...
        L3b * dR(t012);

    % 최종 자코비안
    J = -[J1, J2, J3];
end

== matlab function Model2/Single(Right)_ARM_Simplify/Right_ARM_Real_FK ==
  data: theta input; positions output; ee_pose output
function [positions, ee_pose] = fk_R_3link_explicit(theta)
    L0 = 0.04494;
    L1 = 0.08979;
    L2 = 0.1665;
    L3a = 0.02945;
    L3b = 0.1232;

    t0 = theta(1);
    t1 = theta(2);
    t2 = theta(3);
    t01 = t0 + t1;
    t012 = t01 + t2;

    R = @(theta) [-cos(theta); -sin(theta)];

    P0 = [0; 0];
    P1 = P0 - L0 * R(t0 - pi/2);
    P2 = P1 - L1 * R(t0);
    P3 = P2 - L2 * R(t01);
    P4 = P3 - L3a * R(t012 - pi/2);
    ee_pose = P4 - L3b * R(t012);  % EE 위치
    positions = [P1,P2,P3,P4,ee_pose];
end

== matlab function Model2/Single(Right)_ARM_Simplify/Right_ARM_Real_Simple_FK ==
  data: theta input; positions output; ee_pose output
function [positions, ee_pose] = fk_R_3link_simplify(theta)
    % theta: [theta1, theta2, theta3] (rad)
    % a1, a2, a3: 링크 길이
    % positions: [P0; P1; P2; P3] (각 조인트 위치)
    % ee_pose: [x, y, phi] (EE 위치 + 자세)
    % L0 = 0.04494;
    % L1 = 0.08979;
    % L2 = 0.1665;
    % L3a = 0.02945;
    % L3b = 0.1232;


    offset0 = -atan2(0.04494, 0.08979);
    offset1 = +atan2(0.04494, 0.08979);
    offset2 = -atan2(0.02945, 0.1232);
    offset = 1*[offset0,offset1,offset2]';

    theta = theta + offset;

    L = [sqrt(0.04494^2 + 0.08979^2);
           0.1665;
           sqrt(0.02945^2 + 0.1232^2)];

    theta1 = theta(1);
    theta2 = theta(2);
    theta3 = theta(3);

    % 누적 각도
    t1 = theta1;
    t2 = theta1 + theta2;
    t3 = t2 + theta3;

    % 각 조인트 위치 계산
    P0 = [0; 0];
    P1 = P0 + L(1) * [cos(t1); sin(t1)];
    P2 = P1 + L(2) * [cos(t2); sin(t2)];
    P3 = P2 + L(3) * [cos(t3); sin(t3)];

    % 자세
    phi = t3;

    % 출력
    positions = [P0, P1, P2, P3];  % 각 열이 각 위치
    ee_pose = [P3(1), P3(2)]'; % EE 위치 및 방향
end

== matlab function Model2/Single(Right)_ARM_Simplify/slip_kinematics+Timer1 ==
  settings: updateMethod=DISCRETE
  data: EE_vel_t output; EE_vel_J input; slip_kinematics output; EE_Jaco_start input; elapsedTime input
function [EE_vel_t,slip_kinematics]  = kinema_slip(EE_vel_J,EE_Jaco_start,elapsedTime)


    persistent EE_vel_J_pre lastTime
    if isempty(EE_vel_J_pre)
        EE_vel_J_pre=[0 0]';
        lastTime = elapsedTime;
    end
    
    dt = elapsedTime - lastTime;

    vel_min = -0.005;
    vel_max = 0.005;
    
    dvel_min = -0.005;
    dvel_max = 5e-03;
   

    dEE_vel = EE_vel_J_pre-EE_vel_J;

    EE_vel_t = dEE_vel/dt;
    
    if EE_Jaco_start==1 && all(EE_vel_J >= vel_min & EE_vel_J <= vel_max) && all(EE_vel_t<=dvel_max)
        slip_kinematics =1;
    else
        slip_kinematics=0;
    
    end

    if trackTime(elapsedTime, 1) == 1
        EE_vel_J_pre = EE_vel_J;
        lastTime = elapsedTime;
    end

end

%%
function [flag, del_time] = fcn(data, t)

persistent sw
persistent data_save
persistent tic_time

if isempty(sw)
    sw = 0;
    data_save = 0;
    tic_time = 0;
end

flag = 0;
del_time = 0;

if (data>=0.001)
    if sw == 0
        sw = 1;
        data_save = data;
        tic_time = t;
    end
end

del_t = t - tic_time;

if ((del_t>=1.0) && (sw==1))
    diff_data = abs(data - data_save);
    if diff_data >= 0.1
        flag = 1;
    else
        flag = 0;
    end
    sw = 0;
end


end

== matlab function Model2/Single(Right)_ARM_Simplify/Openning_Motion_Sequence4 ==
  settings: updateMethod=DISCRETE
  data: R_J_Pos input; R_J input; b_flg input; res output; mode output; pos_end_flg input
function [res, mode] = Motion_CMD(R_J_Pos, R_J, b_flg, pos_end_flg)

persistent grip_flg

if isempty(grip_flg)
    grip_flg = 0;
end

deg2rad = pi/180;

R_ee = R_J_Pos(:,4);
R_ee_ = R_ee/norm(R_ee);
R_ee_ = [R_ee_(1), R_ee_(2)]';

Body_Contact_Total = (b_flg(1) == 1) && (b_flg(2) == 1) && (b_flg(3) == 1) && (b_flg(4) == 1);
Pos_End_Total = pos_end_flg;

if (Body_Contact_Total)
    % res = [0 0 0]'*deg2rad;
    % mode = [2 2 2]';
    if grip_flg == 0
        grip_flg = 1;
    end
    R_Jacob = jacobian_fk_R_3link_explicit(R_J);
    res = -pinv(R_Jacob)*(-R_ee_.*[0.1; 0.01]);
    mode = [2 2 2]';
else
    res = [1 2 3]'*deg2rad;
    mode = [2 2 2]';
end

if grip_flg == 1
    R_Jacob = jacobian_fk_R_3link_explicit(R_J);
    res = -pinv(R_Jacob)*[0;0.001];
    mode = [2 2 2]';
end

if Pos_End_Total == 1
    R_Jacob = jacobian_fk_R_3link_explicit(R_J);
    res = -pinv(R_Jacob)*[0;0];
    mode = [2 2 2]';
end
% res = [-45 45 0]'*deg2rad;
% mode = [3 3 3]';


end

function J = jacobian_fk_R_3link_explicit(theta)
    % 링크 길이
    L0 = 0.04494;
    L1 = 0.08979;
    L2 = 0.1665;
    L3a = 0.02945;
    L3b = 0.1232;

    % 조인트 각도
    t0 = theta(1);
    t1 = theta(2);
    t2 = theta(3);

    t01 = t0 + t1;
    t012 = t01 + t2;

    % 편미분 벡터 함수 dR = d/dθ of R(θ)
    dR = @(theta) [sin(theta); -cos(theta)];

    % ∂x/∂theta1
    J1 = ...
        L0 * dR(t0 - pi/2) + ...
        L1 * dR(t0) + ...
        L2 * dR(t01) + ...
        L3a * dR(t012 - pi/2) + ...
        L3b * dR(t012);

    % ∂x/∂theta2
    J2 = ...
        L2 * dR(t01) + ...
        L3a * dR(t012 - pi/2) + ...
        L3b * dR(t012);

    % ∂x/∂theta3
    J3 = ...
        L3a * dR(t012 - pi/2) + ...
        L3b * dR(t012);

    % 최종 자코비안
    J = -[J1, J2, J3];
end

== matlab function Model2/Single(Right)_ARM_Simplify/End_Position_Flg ==
  data: res output; R_J input
function res  = End_Flag_Maker( R_J  )

deg2rad = 0.017453292519943;
rad2deg = 57.295779513082323;

R_END_FLG = 0;

Limit_Angle0 =     9.425*deg2rad;
Limit_Angle1 =   71.133*deg2rad;
Limit_Angle2 = 106.792*deg2rad;

R_END_FLG = End_Checker(R_J, [-Limit_Angle0,Limit_Angle1,Limit_Angle2]);

res = R_END_FLG;

end

function res = End_Checker (Joint_Angle, Limit_Angle)

Limit_J0 = Limit_Angle(1);
Limit_J1 = Limit_Angle(2);
Limit_J2 = Limit_Angle(3);

J0 = Joint_Angle(1);
J1 = Joint_Angle(2);
J2 = Joint_Angle(3);

del = 5*pi/180;

J0_flg = 0; J1_flg = 0; J2_flg = 0;

if ((J0 <= (Limit_J0+del)) && (J0 >= (Limit_J0-del)))
    J0_flg = 1;
else
    J0_flg = 0;
end

if ((J1 <= (Limit_J1+del)) && (J1 >= (Limit_J1-del)))
    J1_flg = 1;
else
    J1_flg = 0;
end

if ((J2 <= (Limit_J2+del)) && (J2 >= (Limit_J2-del)))
    J2_flg = 1;
else
    J2_flg = 0;
end

if (J0_flg && J1_flg && J2_flg)
    res = 1;
else
    res = 0;
end

end

== matlab function Model2/Quad_ARM_Simplify/Down_ARM/MATLAB Function2 ==
  settings: updateMethod=DISCRETE
  data: cmd input; t_cmd output; cmd_d input; t_mea input; vd_mea input; v_mea input; p_mea input; mode input; tc_gain input; vc_gain input; pc_gain input; dt input
function t_cmd = motor_control(cmd, cmd_d, t_mea, vd_mea, v_mea, p_mea, mode, tc_gain, vc_gain, pc_gain, dt)

persistent I_save
persistent first_flg

if isempty(first_flg)
    I_save = 0;
    first_flg = 1;
end

if(mode == 1)%torque control
    % cmd : torque command [Nm]
    kp = tc_gain(1);
    ki = tc_gain(2);
    err = cmd - t_mea;
    t_cmd = kp*(cmd - t_mea) + ki*I_save;
    I_save = I_save + err*dt;

elseif(mode == 2) %velocity control
    % cmd : velocity command [rad/s]
    kp = vc_gain(1);
    % ki = vc_gain(2);
    kd = vc_gain(3);

    err = cmd - v_mea;
    errd = cmd_d - vd_mea;
    % t_cmd = (kp*err) + (kd*errd);
    t_cmd = (kp*err) + (kd*errd);
elseif(mode == 3) %position control : position command [rad]
    kp = pc_gain(1);
    % ki = pc_gain(2);
    kd = pc_gain(3);

    err = cmd - p_mea;
    errd = cmd_d - v_mea;
    t_cmd = (kp*err) + (kd*errd);
else%torque control
    t_cmd = 0;
end



end

== matlab function Model2/Quad_ARM_Simplify/Down_ARM/MATLAB Function3 ==
  data: v_sig input; v_out output; vd_out output; vd_sig input; t_mea input
function [v_out, vd_out] = limit_checker(v_sig,vd_sig,  t_mea)


if(abs(t_mea)>=0.01)
    vd_out = 0;
    v_out = 0;
else
    vd_out = vd_sig;
    v_out = v_sig;
end




end

== matlab function Model2/Single_ARM/MATLAB Function1 ==
  data: theta input; J output
function J = jacobian_3link(theta)
    L0 = 0.04494;
    L1 = 0.08979;
    L2 = 0.1665;
    L3a = 0.02945;
    L3b = 0.1232;

    t0 = theta(1);
    t1 = theta(2);
    t2 = theta(3);
    t01 = t0 + t1;
    t012 = t01 + t2;

    Rp = @(theta) [-sin(theta); cos(theta)]; 

    J1 =  L0 * Rp(t0 + pi/2) ...
         +L1 * Rp(t0) ...
         +L2 * Rp(t01) ...
         +L3a * Rp(t012 + pi/2) ...
         +L3b * Rp(t012);

    J2 =  L2 * Rp(t01) ...
         +L3a * Rp(t012 + pi/2) ...
         +L3b * Rp(t012);

    J3 =  L3a * Rp(t012 + pi/2) ...
         +L3b * Rp(t012);

    J = [J1, J2, J3];
end

== matlab function Model2/Quad_ARM_Simplify/Down_ARM/MATLAB Function4 ==
  settings: updateMethod=DISCRETE
  data: cmd input; t_cmd output; cmd_d input; t_mea input; vd_mea input; v_mea input; p_mea input; mode input; tc_gain input; vc_gain input; pc_gain input; dt input
function t_cmd = motor_control(cmd,cmd_d, t_mea, vd_mea, v_mea, p_mea, mode, tc_gain, vc_gain, pc_gain, dt)

persistent I_save
persistent first_flg

if isempty(first_flg)
    I_save = 0;
    first_flg = 1;
end

if(mode == 1)%torque control
    % cmd : torque command [Nm]
    kp = tc_gain(1);
    ki = tc_gain(2);
    err = cmd - t_mea;
    t_cmd = kp*(cmd - t_mea) + ki*I_save;
    I_save = I_save + err*dt;

elseif(mode == 2) %velocity control
    % cmd : velocity command [rad/s]
    kp = vc_gain(1);
    % ki = vc_gain(2);
    kd = vc_gain(3);

    err = cmd - v_mea;
    errd = cmd_d - vd_mea;
    % t_cmd = (kp*err) + (kd*errd);
    t_cmd = (kp*err) + (kd*errd);
elseif(mode == 3) %position control : position command [rad]
    kp = pc_gain(1);
    ki = pc_gain(2);
    kd = pc_gain(3);

    err = cmd - p_mea;
    errd = cmd_d - v_mea;
    t_cmd = (kp*err) + (kd*errd);
else%torque control
    t_cmd = 0;
end



end

== matlab function Model2/Quad_ARM_Simplify/Down_ARM/MATLAB Function5 ==
  data: v_sig input; v_out output; vd_out output; vd_sig input; t_mea input
function [v_out, vd_out] = limit_checker(v_sig,vd_sig,  t_mea)


if(abs(t_mea)>=0.01)
    vd_out = 0;
    v_out = 0;
else
    vd_out = vd_sig;
    v_out = v_sig;
end




end
